simulink model "controlled_rectifier_with_filter_r2016b1"  (Simulink 8.8)
settings: Solver=ode8  StartTime=0.0  StopTime=0.3  FixedStep=2e-6  RelTol=1e-3
undefined symbols (not defined in the file or in its folder): D1, Delta, powergui, spspowerguiLib
libraries: spsThyristorLib x6, simulink x3, spsVoltageMeasurementLib x3, spsSeriesRLCBranchLib x2, spsThreePhaseVIMeasurementLib x2, spsCurrentMeasurementLib x1, spsSawtoothGeneratorLib x1, spsSeriesRLCLoadLib x1, spsThreePhaseTransformerTwoWindingsLib x1, spsThreePhaseSourceLib x1
settings Model: Creator=Aditya  LastModifiedBy=Aditya
settings DataIOCC: LimitDataPoints=off  SaveFormat=Dataset  SignalLoggingSaveFormat=Dataset  ReturnWorkspaceOutputs=on
settings OptimizationCC: LifeSpan=auto
settings DebuggingCC: UnderspecifiedInitializationDetection=Simplified  MergeDetectMultiDrivingBlocksExec=error  FcnCallInpInsideContextMsg=error  StateNameClashWarn=none  SFUnexpectedBacktrackingDiag=error  SFNoUnconditionalDefaultTransitionDiag=error  SFExecutionAtInitializationDiag=warning  SFMachineParentedDataDiag=error
settings HardwareCC: ProdBitPerPointer=64  ProdBitPerSizeT=64  ProdBitPerPtrDiffT=64  ProdLargestAtomicFloat=Float  ProdIntDivRoundTo=Zero  ProdEndianess=LittleEndian  ProdWordSize=64  ProdHWDeviceType=Intel->x86-64 (Windows64)
settings ModelReferenceCC: PropagateSignalLabelsOutOfModel=on
settings SFSimCC: SimUseLocalCustomCode=on
settings RTWCC: RTWUseLocalCustomCode=on
settings GRTTargetCC: TargetLangStandard=C99 (ISO)  CombineOutputUpdateFcns=on  GRTInterface=off
settings ConfigComp: CovMetricSettings=dwe  CovSaveCumulativeToWorkspaceVar=off  CovSaveSingleToWorkspaceVar=off  CovExternalEMLEnable=on

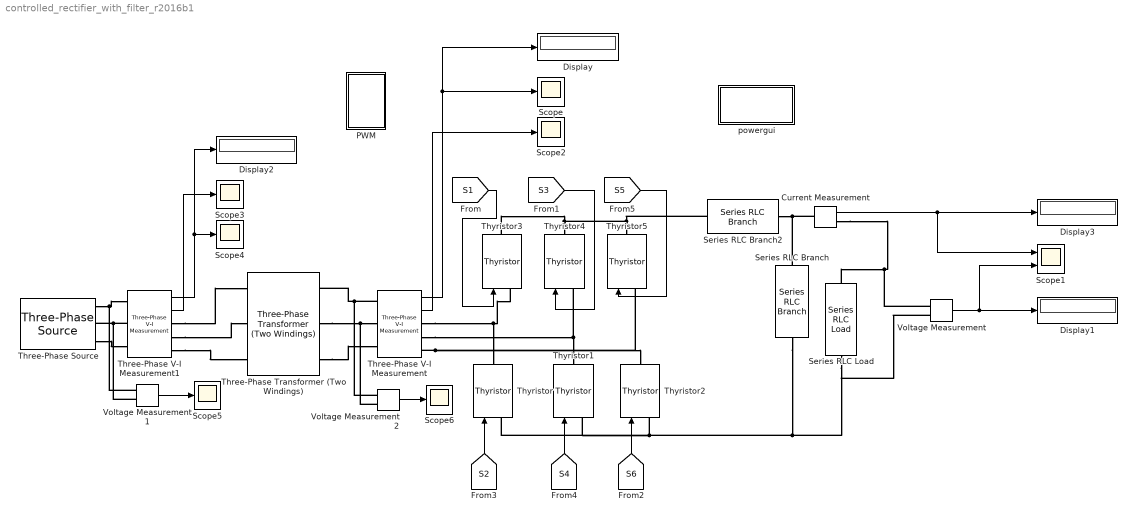
== system controlled_rectifier_with_filter_r2016b1 ==
  Current Measurement : spsCurrentMeasurementLib/Current Measurement  PhasorSimulation=off  OutputType=Complex  PSBequivalent=0
  Display{,1..3} (4 alike) : Display
  PWM : Subsystem
  Scope{,2..6} (6 alike) : Scope
  Scope1 : Scope  NumInputPorts=2
  Series RLC Branch : spsSeriesRLCBranchLib/Series RLC Branch  LConnTagsString=__new0  RConnTagsString=__new0  BranchType=C  Resistance=1  Inductance=1e-3  SetiL0=off  InitialCurrent=0  Capacitance=470e-6  Setx0=off  InitialVoltage=0  Measurements=None
  Series RLC Branch2 : spsSeriesRLCBranchLib/Series RLC Branch  LConnTagsString=__new0  RConnTagsString=__new0  BranchType=RL  Resistance=15  Inductance=25e-3  SetiL0=off  InitialCurrent=0  Capacitance=1e-6  Setx0=off  InitialVoltage=0  Measurements=None
  Series RLC Load : spsSeriesRLCLoadLib/Series RLC Load  LConnTagsString=a  RConnTagsString=__new0  NominalVoltage=370  NominalFrequency=50  ActivePower=1e3  InductivePower=0.8e3  CapacitivePower=0  Setx0=off  InitialVoltage=0  SetiL0=off  InitialCurrent=0  Measurements=None  LoadType=constant Z
  Three-Phase Transformer (Two Windings) : spsThreePhaseTransformerTwoWindingsLib/Three-Phase Transformer (Two Windings)  Winding1Connection=Delta (D1)  Winding2Connection=Yg  CoreType=Three single-phase transformers  SetSaturation=off  Hysteresis=off  DataFile='hysteresis'  SetInitialFlux=off  Measurements=None  UNITS=SI  NominalPower=[ 1.5e3 , 50 ]  Winding1=[25000 50 0.66315]  Winding2=[415 0.0864 0.0011459]  Rm=2.5e+06  Lm=6631.5  L0=0.5  Saturation=[0 0;0.66653 1910.3;277.72 2419.7]  InitialFluxes=[ 0.8 , -0.8 , 0.7 ]  BreakLoop=off  DiscreteSolver=Trapezoidal iterative  DataType=on  TransfoNumber=1
  Three-Phase V-I Measurement : spsThreePhaseVIMeasurementLib/Three-Phase V-I Measurement  VoltageMeasurement=phase-to-phase  SetLabelV=off  LabelV=Vabc  Vpu=off  VpuLL=off  CurrentMeasurement=yes  SetLabelI=off  LabelI=Iabc  Ipu=off  Pbase=100e6  Vbase=500e3  OutputType=Complex  PhasorSimulation=off  PSBequivalent=0
  Three-Phase V-I Measurement1 : spsThreePhaseVIMeasurementLib/Three-Phase V-I Measurement  VoltageMeasurement=phase-to-phase  SetLabelV=off  LabelV=Vabc  Vpu=off  VpuLL=off  CurrentMeasurement=yes  SetLabelI=off  LabelI=Iabc  Ipu=off  Pbase=100e6  Vbase=500e3  OutputType=Complex  PhasorSimulation=off  PSBequivalent=0
  Three-Phase Source : spsThreePhaseSourceLib/Three-Phase Source  InternalConnection=Yg  VoltagePhases=off  Voltage=25e3  PhaseAngle=0  Voltage_phases=[25e3 25e3 25e3]/sqrt(3)  PhaseAngles_phases=[0 -120 +120]  Frequency=50  NonIdealSource=on  SpecifyImpedance=off  Resistance=0.8929  Inductance=16.58e-3  ShortCircuitLevel=100e6  BaseVoltage=25e3  XRratio=7  BusType=PV  Pref=50e3  Qref=0  Prefabc=[10e3, 10e3, 10e3]  Qrefabc=[0, 0, 0]  Qmin=-inf  Qmax=inf
  Thyristor{,1..5} (6 alike) : spsThyristorLib/Thyristor  Ron=0.001  Lon=0  Vf=0.8  IC=0  Rs=500  Cs=250e-9  Measurements=off
  Voltage Measurement : spsVoltageMeasurementLib/Voltage Measurement  PhasorSimulation=off  OutputType=Complex  PSBequivalent=0
  Voltage Measurement1 : spsVoltageMeasurementLib/Voltage Measurement  PhasorSimulation=off  OutputType=Complex  PSBequivalent=0
  Voltage Measurement2 : spsVoltageMeasurementLib/Voltage Measurement  PhasorSimulation=off  OutputType=Complex  PSBequivalent=0
  powergui : Subsystem  Priority=1  AncestorBlock=spspowerguiLib/powergui  DialogController=POWERSYS.PowerSysDialog  InitFcn=powergui( 'InitFcn_Callback' , gcb , 0 , [ ] );  mask(PSB option menu block){SimulationMode=Discrete, SampleTime=2e-6, frequency=60, Iterations=50, frequencyindice=50, Pbase=100e6, ErrMax=1e-4, UnitsV=kV, UnitsW=MW, buscounter=0, FunctionMessages=off, echomessages=off, EnableUseOfTLC=off, CurrentSourceSwitches=off, DisableSnubberDevices=off, DisableRonSwitches=off, DisableVfSwitches=off, DisplayEquations=off, AutomaticDiscreteSolvers=off, SolverType=Tustin/Backward Euler (TBE), Interpol=off, ExternalGateDelay=off, methode=off, Ts=100, x0status=blocks, SPID=on, SwTol=0, HookPort=off, NonlinearTolerance=1e-4, nMaxIteration=100, ContinueOnMaxIteration=off, RestoreLinks=warning, ResistiveCurrentMeasurement=off, Frange=[0:2:500], Ylog=off, Xlog=on, ShowGrid=off, save=off, variable=ZData, structure=0, ZoomFFT=off, StartTime=0.0, cycles=1, DisplayStyle=1, fundamental=60, FreqAxis=off, MaxFrequency=1000, frequencyindicesteady=1, RmsSteady=1, display=off}
      mask prompts: SimulationMode "Simulation type:"; SampleTime "Sample time (s):"; frequency "Frequency (Hz):"; Iterations "Max iterations"; frequencyindice "Frequency (Hz)"; Pbase "Base power (VA)"; ErrMax "PQ tolerance (pu)"; UnitsV "Voltage units"; UnitsW "Power units"; buscounter "Load flow bus counter"; FunctionMessages "Disable Specialized Power Systems warnings"; echomessages "Display Specialized Power Systems compilation messages"; EnableUseOfTLC "Use TLC file when in Accelerator Simulation Mode and for code generation"; CurrentSourceSwitches "Disable ideal switching"; DisableSnubberDevices "Disable snubbers in switching devices"; DisableRonSwitches "Disable Ron resistances in switching devices"; DisableVfSwitches "Disable forward voltages in switching devices"; DisplayEquations "Display circuit differential equations"; AutomaticDiscreteSolvers "Automatically handle Discrete solver and Advanced tab solver settings of blocks"; SolverType "Discrete solver"; Interpol "Interpolate switching events"; ExternalGateDelay "Use time-stamped gate signals"; methode "Store switching topologies"; Ts "Buffer size (MBytes):"; x0status "Start simulation with initial electrical states from:"; SPID "Use ideal switching devices"; SwTol "Switch tolerance"; HookPort "Allow multiple powergui blocks"; NonlinearTolerance "Solver tolerance"; nMaxIteration "Maximum number of iterations"; ContinueOnMaxIteration "Continue Simulation if maximum number of iterations is reached"; RestoreLinks "Restore disabled links of Simscape Power Systems ST blocks:"; ResistiveCurrentMeasurement "Use non ideal current measurement blocks (1e-4Ohm internal resistance)"; Frange "Frequency Range"; Ylog "Log impedance"; Xlog "log Frequency"; ShowGrid "grid"; save "Save Data To Workspace"; variable "Variable Name"; structure "Structure Name (PSBFFTSCOPE)"; ZoomFFT "ZoomFFT (PSBFFTSCOPE)"; StartTime "Start Time (PSBFFTSCOPE)"; cycles "Cycles (PSBFFTSCOPE)"; DisplayStyle "Display style (PSBFFTSCOPE)"; fundamental "Fundamental (PSBFFTSCOPE)"; FreqAxis "Frequency Axis (PSBFFTSCOPE)"; MaxFrequency "Max Frequency (PSBFFTSCOPE)"; frequencyindicesteady "Frequency indice (STEADYSTATE)"; RmsSteady "RMS display (STEADYSTATE)"; display "Display Results"
      mask help: Set simulation type, simulation parameters, and preferences.
      mask init:
      | dispMessage = powergui('MaskInitialization',gcb,SimulationMode,SampleTime);
      settings: PreSaveFcn=powergui( 'PreSaveFcn_Callback' , gcb , [ ] , [ ] );  OpenFcn=sps_rtmsupport('OpenFcn',gcbh)
      mask Help: helpview(psbhelp)
      mask TypeOptions SimulationMode: Continuous | Discrete | Phasor | Discrete phasor
      mask Callback SimulationMode: powergui('SimulationType',[],[],gcb);
      mask TypeOptions UnitsV: V | kV
      mask TypeOptions UnitsW: W | kW | MW
      mask Callback CurrentSourceSwitches: powergui('SimulationType',[],[],gcb);
      mask Callback AutomaticDiscreteSolvers: powergui('SimulationType',[],[],gcb);
      mask TypeOptions SolverType: Tustin/Backward Euler (TBE) | Tustin | Backward Euler
      mask Callback SolverType: powergui('SimulationType',[],[],gcb);
      mask Callback Interpol: powergui('SimulationType',[],[],gcb);
      mask Callback ExternalGateDelay: powergui('SimulationType',[],[],gcb);
      mask Callback methode: powergui('SimulationType',[],[],gcb);
      mask TypeOptions x0status: blocks | steady | zero
      mask TypeOptions RestoreLinks: yes | warning | no
      mask Callback display: sps_rtmsupport('parametereditingmodes',gcbh) % Will be executed last in parameter callbacks to ensure mask enable consistency
      mask DialogControl AutoSolverNote Prompt: The Simulation type parameter is governed by Simulink. To access the Powergui solver settings, unselect auto (Automatic solver selection) solver in the Simulink solver options.
      mask DialogControl StateAnalyzer Prompt: Measurements and States Analyzer
      mask DialogControl StateAnalyzer Callback: powerStates(bdroot(gcb))
      mask DialogControl RLCLineParameters Prompt: Power Line Parameters
      mask DialogControl RLCLineParameters Callback:
      | close_system(gcb)
      | powerLineParameters
      mask DialogControl DecouplingLines Prompt: Specify Decoupling Lines
      mask DialogControl DecouplingLines Tooltip: Click to replace selected Distributed Parameters Line blocks with Decoupling Line blocks
      mask DialogControl DecouplingLines Callback:
      | close_system(gcb);
      | DecouplingLineReplace(gcs)
      mask DialogControl LoadFlow Prompt: Load Flow Analyzer
      mask DialogControl LoadFlow Callback:
      | close_system(gcb)
      | powerLoadFlow
      mask DialogControl Container11 Prompt: Load Flow Parameters
      mask DialogControl MachineInitialization Prompt: Machine Initialization
      mask DialogControl MachineInitialization Callback:
      | close_system(gcb)
      | powericon('machineInitTool',bdroot(gcb),gcb)
      mask DialogControl ImpedanceMeasurement Prompt: Impedance Measurement
      mask DialogControl ImpedanceMeasurement Callback:
      | close_system(gcb)
      | power_zmeter(bdroot(gcb),gcb)
      mask DialogControl FFTAnalysis Prompt: FFT Analysis
      mask DialogControl FFTAnalysis Callback:
      | close_system(gcb)
      | power_fftscope(bdroot(gcb),gcb)
      mask DialogControl LinearSystemAnalyzer Prompt: Use Linear System Analyzer
      mask DialogControl LinearSystemAnalyzer Callback:
      | close_system(gcb)
      | power_ltiview(bdroot(gcb),gcb)
      mask DialogControl HysteresisDesign Prompt: Hysteresis Design
      mask DialogControl HysteresisDesign Callback:
      | close_system(gcb)
      | power_hysteresis(bdroot(gcb),gcb)
      mask DialogControl Control14 Prompt: Customize SPS blocks
      mask DialogControl Control14 Callback:
      | close_system(gcb);
      | power_customize;
      mask DialogControl GenerateReprot Prompt: Generate Report
      mask DialogControl GenerateReprot Callback:
      | close_system(gcb)
      | power_report(bdroot(gcb),gcb)
      mask DialogControl Solver Prompt: Solver
      mask DialogControl SolverDetails Prompt: Solver details for nonlinear elements
      mask Display: color('blue'),disp(dispMessage)
  wires:
  Three-Phase V-I Measurement/1 -> Scope/1, Display/1
  Three-Phase V-I Measurement/2 -> Scope2/1
  Voltage Measurement/1 -> Scope1/2, Display1/1
  Current Measurement/1 -> Display3/1, Scope1/1
  Three-Phase V-I Measurement1/1 -> Scope4/1, Display2/1
  Three-Phase V-I Measurement1/2 -> Scope3/1
  Voltage Measurement1/1 -> Scope5/1
  Voltage Measurement2/1 -> Scope6/1
  [S2] -> Thyristor/1
  [S4] -> Thyristor1/1
  [S6] -> Thyristor2/1
  [S1] -> Thyristor3/1
  [S3] -> Thyristor4/1
  [S5] -> Thyristor5/1
  connections:
  Three-Phase V-I Measurement/LConn1 -- Three-Phase Transformer (Two Windings)/RConn1 -- Voltage Measurement2/LConn1
  Three-Phase Transformer (Two Windings)/RConn2 -- Voltage Measurement2/LConn2 -- Three-Phase V-I Measurement/LConn2
  Three-Phase Transformer (Two Windings)/RConn3 -- Three-Phase V-I Measurement/LConn3
  Three-Phase V-I Measurement/RConn1 -- Thyristor3/LConn1 -- Thyristor/RConn1
  Three-Phase V-I Measurement/RConn2 -- Thyristor1/RConn1 -- Thyristor4/LConn1
  Three-Phase V-I Measurement/RConn3 -- Thyristor2/RConn1 -- Thyristor5/LConn1
  Thyristor1/LConn1 -- Thyristor/LConn1 -- Voltage Measurement/LConn2 -- Series RLC Load/LConn1 -- Series RLC Branch/RConn1 -- Thyristor2/LConn1
  Current Measurement/RConn1 -- Series RLC Load/RConn1 -- Voltage Measurement/LConn1
  Three-Phase V-I Measurement1/LConn2 -- Voltage Measurement1/LConn2 -- Three-Phase Source/RConn2
  Three-Phase Source/RConn1 -- Voltage Measurement1/LConn1 -- Three-Phase V-I Measurement1/LConn1
  Three-Phase Source/RConn3 -- Three-Phase V-I Measurement1/LConn3
  Three-Phase V-I Measurement1/RConn1 -- Three-Phase Transformer (Two Windings)/LConn1
  Three-Phase V-I Measurement1/RConn2 -- Three-Phase Transformer (Two Windings)/LConn2
  Three-Phase V-I Measurement1/RConn3 -- Three-Phase Transformer (Two Windings)/LConn3
  Thyristor5/RConn1 -- Series RLC Branch2/LConn1 -- Thyristor3/RConn1 -- Thyristor4/RConn1
  Current Measurement/LConn1 -- Series RLC Branch2/RConn1 -- Series RLC Branch/LConn1

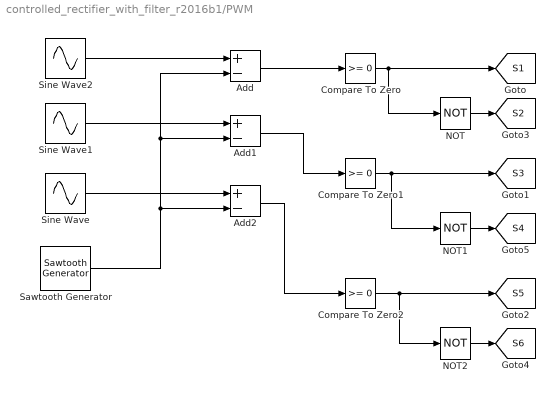
== system controlled_rectifier_with_filter_r2016b1/PWM ==
  Add : Sum  Inputs=+-
  Add1 : Sum  Inputs=+-
  Add2 : Sum  Inputs=+-
  Compare To Zero : simulink/Logic and Bit Operations/Compare To Zero  relop=>=  OutDataTypeStr=boolean
  Compare To Zero1 : simulink/Logic and Bit Operations/Compare To Zero  relop=>=  OutDataTypeStr=boolean
  Compare To Zero2 : simulink/Logic and Bit Operations/Compare To Zero  relop=>=  OutDataTypeStr=boolean
  NOT : Logic  Operator=NOT  IconShape=distinctive  AllPortsSameDT=off  OutDataTypeStr=boolean
  NOT1 : Logic  Operator=NOT  IconShape=distinctive  AllPortsSameDT=off  OutDataTypeStr=boolean
  NOT2 : Logic  Operator=NOT  IconShape=distinctive  AllPortsSameDT=off  OutDataTypeStr=boolean
  Sawtooth Generator : spsSawtoothGeneratorLib/Sawtooth Generator  Freq=1e03  Phase=0  Ts=0
  Sine Wave : Sin  Frequency=2*pi*50  Phase=(-2*pi/3)+pi/6  SampleTime=0
  Sine Wave1 : Sin  Frequency=2*pi*50  Phase=(2*pi/3)+pi/6  SampleTime=0
  Sine Wave2 : Sin  Frequency=2*pi*50  Phase=pi/6  SampleTime=0
  tag scope: S1=global, S2=global, S3=global, S4=global, S5=global, S6=global
  wires:
  Sine Wave/1 -> Add2/1
  Sawtooth Generator/1 -> Add2/2, Add1/2, Add/2
  Compare To Zero/1 -> NOT/1, [S1]
  Sine Wave2/1 -> Add/1
  Compare To Zero2/1 -> NOT2/1, [S5]
  Compare To Zero1/1 -> NOT1/1, [S3]
  NOT2/1 -> [S6]
  Sine Wave1/1 -> Add1/1
  NOT/1 -> [S2]
  Add1/1 -> Compare To Zero1/1
  Add/1 -> Compare To Zero/1
  Add2/1 -> Compare To Zero2/1
  NOT1/1 -> [S4]

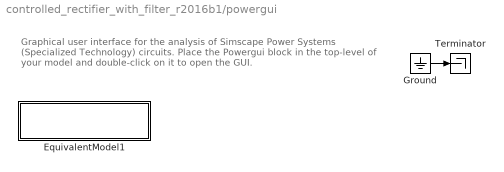
== system controlled_rectifier_with_filter_r2016b1/powergui ==
  note: Graphical user interface for the analysis of
      | Simscape Power Systems (Specialized Technology) circuits.
      | Place the Powergui block in the top-level of your model and double-click
      | on it to open the GUI.
  EquivalentModel1 : Subsystem
      mask init:
      | S  = GetDataForEquivalentModel('Discrete',gcbh);
      mask Display:
      | color('red')
      | disp('EQUIVALENT CIRCUIT\nDiscrete')
  Ground : Ground
  Terminator : Terminator
  wires:
  Ground/1 -> Terminator/1

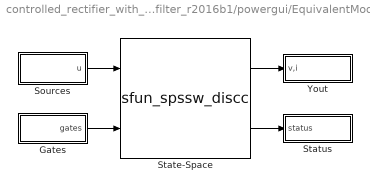
== system controlled_rectifier_with_filter_r2016b1/powergui/EquivalentModel1 ==
  Gates : Subsystem
  Sources : Subsystem
  State-Space : S-Function  FunctionName=sfun_spssw_discc  Parameters=S.Ts,S.A, S.B, S.C, S.D, S.x0, S.EnableUseOfTLC,S.SwitchResistance ,S.SwitchType, S.SwitchGateInitialValue, S.OutputsToResetToZero, S.TBEON,S.SaveMatrices,S.BufferSize  SFunctionDeploymentMode=off  EnableBusSupport=off
  Status : Subsystem
  Yout : Subsystem
  wires:
  Gates/1(gates) -> State-Space/2
  Sources/1(u) -> State-Space/1
  State-Space/2 -> Status/1(status)
  State-Space/1 -> Yout/1(v,i)

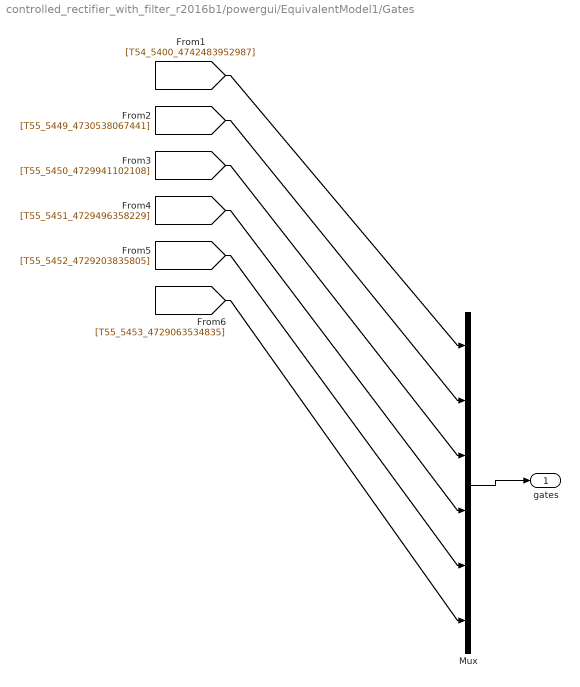
== system controlled_rectifier_with_filter_r2016b1/powergui/EquivalentModel1/Gates ==
  Mux : Mux  Inputs=[1 1 1 1 1 1]
  gates : Outport
  wires:
  Mux/1 -> gates/1
  [T54_5400_4742483952987] -> Mux/1
  [T55_5449_4730538067441] -> Mux/2
  [T55_5450_4729941102108] -> Mux/3
  [T55_5451_4729496358229] -> Mux/4
  [T55_5452_4729203835805] -> Mux/5
  [T55_5453_4729063534835] -> Mux/6

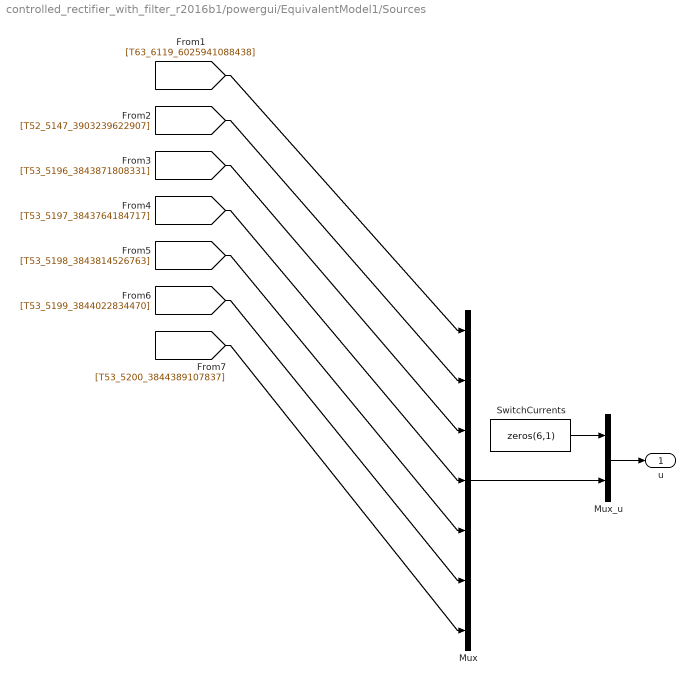
== system controlled_rectifier_with_filter_r2016b1/powergui/EquivalentModel1/Sources ==
  Mux : Mux  Inputs=[3 1 1 1 1 1 1]
  Mux_u : Mux  Inputs=[6 9]
  SwitchCurrents : Constant  Value=zeros(6,1)
  u : Outport
  wires:
  Mux_u/1 -> u/1
  SwitchCurrents/1 -> Mux_u/1
  Mux/1 -> Mux_u/2
  [T63_6119_6025941088438] -> Mux/1
  [T52_5147_3903239622907] -> Mux/2
  [T53_5196_3843871808331] -> Mux/3
  [T53_5197_3843764184717] -> Mux/4
  [T53_5198_3843814526763] -> Mux/5
  [T53_5199_3844022834470] -> Mux/6
  [T53_5200_3844389107837] -> Mux/7

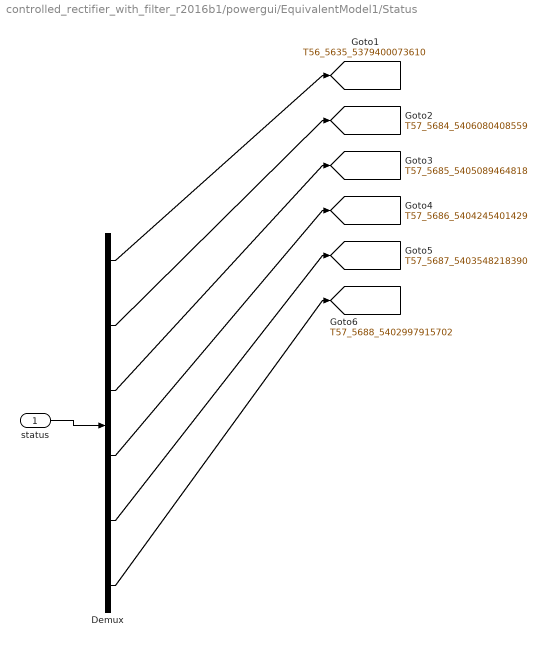
== system controlled_rectifier_with_filter_r2016b1/powergui/EquivalentModel1/Status ==
  status : Inport
  Demux : Demux  Outputs=[1 1 1 1 1 1]
  tag scope: T56_5635_5379400073610=global, T57_5684_5406080408559=global, T57_5685_5405089464818=global, T57_5686_5404245401429=global, T57_5687_5403548218390=global, T57_5688_5402997915702=global
  wires:
  status/1 -> Demux/1
  Demux/1 -> [T56_5635_5379400073610]
  Demux/2 -> [T57_5684_5406080408559]
  Demux/3 -> [T57_5685_5405089464818]
  Demux/4 -> [T57_5686_5404245401429]
  Demux/5 -> [T57_5687_5403548218390]
  Demux/6 -> [T57_5688_5402997915702]

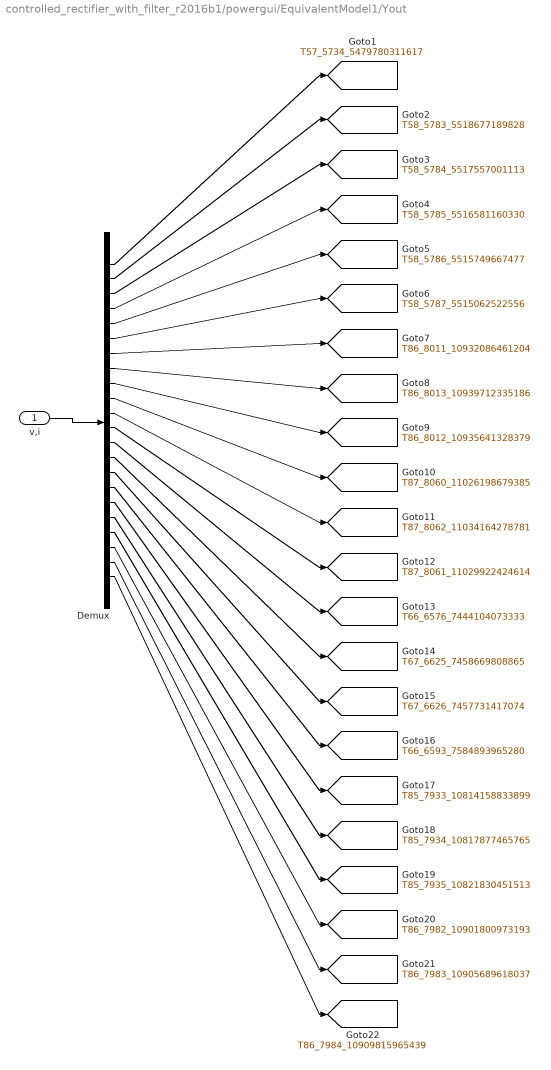
== system controlled_rectifier_with_filter_r2016b1/powergui/EquivalentModel1/Yout ==
  v,i : Inport
  Demux : Demux  Outputs=[1 1 1 1 1 1 1 1 1 1 1 1 1 1 1 1 1 1 1 1 1 1]
  tag scope: T57_5734_5479780311617=global, T58_5783_5518677189828=global, T58_5784_5517557001113=global, T58_5785_5516581160330=global, T58_5786_5515749667477=global, T58_5787_5515062522556=global, T66_6576_7444104073333=global, T66_6593_7584893965280=global, T67_6625_7458669808865=global, T67_6626_7457731417074=global, T85_7933_10814158833899=global, T85_7934_10817877465765=global, T85_7935_10821830451513=global, T86_7982_10901800973193=global, T86_7983_10905689618037=global, T86_7984_10909815965439=global, T86_8011_10932086461204=global, T86_8012_10935641328379=global, T86_8013_10939712335186=global, T87_8060_11026198679385=global, T87_8061_11029922424614=global, T87_8062_11034164278781=global
  wires:
  v,i/1 -> Demux/1
  Demux/1 -> [T57_5734_5479780311617]
  Demux/2 -> [T58_5783_5518677189828]
  Demux/3 -> [T58_5784_5517557001113]
  Demux/4 -> [T58_5785_5516581160330]
  Demux/5 -> [T58_5786_5515749667477]
  Demux/6 -> [T58_5787_5515062522556]
  Demux/7 -> [T86_8011_10932086461204]
  Demux/8 -> [T86_8013_10939712335186]
  Demux/9 -> [T86_8012_10935641328379]
  Demux/10 -> [T87_8060_11026198679385]
  Demux/11 -> [T87_8062_11034164278781]
  Demux/12 -> [T87_8061_11029922424614]
  Demux/13 -> [T66_6576_7444104073333]
  Demux/14 -> [T67_6625_7458669808865]
  Demux/15 -> [T67_6626_7457731417074]
  Demux/16 -> [T66_6593_7584893965280]
  Demux/17 -> [T85_7933_10814158833899]
  Demux/18 -> [T85_7934_10817877465765]
  Demux/19 -> [T85_7935_10821830451513]
  Demux/20 -> [T86_7982_10901800973193]
  Demux/21 -> [T86_7983_10905689618037]
  Demux/22 -> [T86_7984_10909815965439]
